simulink model "VVI"  (R2020a)
settings: Solver=FixedStepAuto  StartTime=0.0  StopTime=inf  FixedStep=0.001  RelTol=1e-3  EnableMultiTasking=on
undefined symbols (not defined in the file): D1, D10, D11, D12, D13, D2, D3, D4, D5, D7, D8, D9, PTA0, PTA1, PTA2, PTB23, PTB9, PTC17, PTC3, PTC4, PTD0, PTD1, PTD2, PTD3
libraries: frdmk64flib x12
settings Model: ExtModeTrigDuration=5  Creator=12268  LastModifiedBy=12268
settings OptimizationCC: EnhancedBackFolding=on  PassReuseOutputArgsAs=Individual arguments  ZeroExternalMemoryAtStartup=off  ZeroInternalMemoryAtStartup=off  MaxStackSize=64  OptimizeBlockOrder=speed  DifferentSizesBufferReuse=on  OptimizationCustomize=off  EfficientTunableParamExpr=on
settings DebuggingCC: ParameterTunabilityLossMsg=error
settings HardwareCC: ProdBitPerPointer=32  ProdBitPerSizeT=32  ProdBitPerPtrDiffT=32  ProdLargestAtomicInteger=Long  ProdLargestAtomicFloat=Double  ProdWordSize=32  ProdHWDeviceType=ARM Compatible->ARM Cortex
settings SFSimCC: MATLABDynamicMemAlloc=off
settings RTWCC: SystemTargetFile=ert.tlc  HardwareBoard=NXP FRDM-K64F  TemplateMakefile=ert_default_tmf  Toolchain=GNU Tools for ARM Embedded Processors
settings CodeAppCC: ForceParamTrailComments=on  IgnoreCustomStorageClasses=off  OperatorAnnotations=on  SimulinkDataObjDesc=on  SFDataObjDesc=on  InsertBlockDesc=on

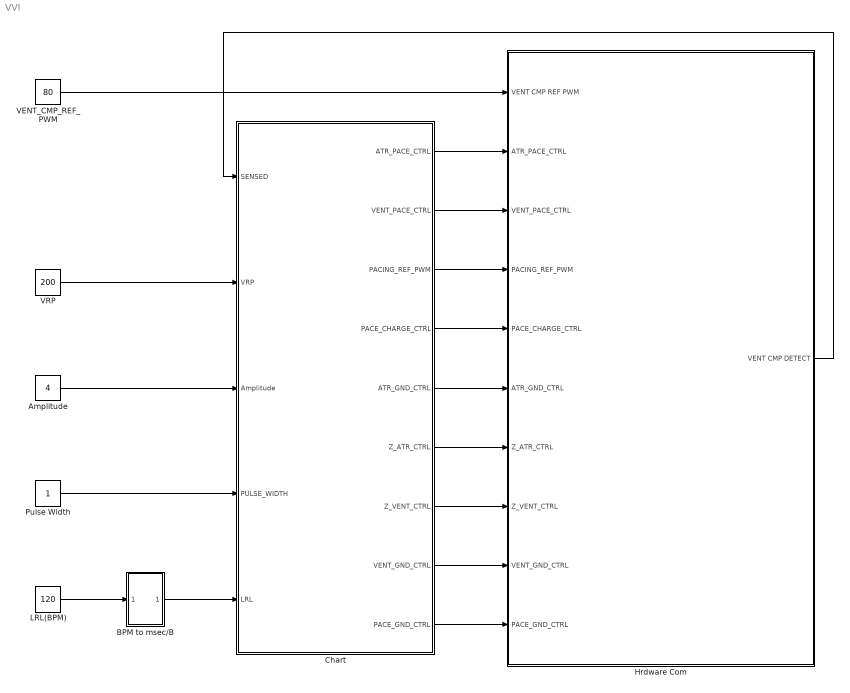
== system VVI ==
  Amplitude : Constant  Value=4  OutDataTypeStr=double
  "BPM to msec/B " : Subsystem
  Chart : Stateflow chart  TreatAsAtomicUnit=on
  Hrdware Com : Subsystem
  LRL(BPM) : Constant  Value=120  OutDataTypeStr=double
  Pulse Width : Constant  OutDataTypeStr=uint16
  VENT_CMP_REF_PWM : Constant  Value=80  OutDataTypeStr=double
  VRP : Constant  Value=200  OutDataTypeStr=uint16
  wires:
  Amplitude/1 -> Chart/3(Amplitude)
  LRL(BPM)/1 -> "BPM to msec/B "/1(In1)
  Pulse Width/1 -> Chart/4(PULSE_WIDTH)
  "BPM to msec/B "/1(Out1) -> Chart/5(LRL)
  Chart/1(ATR_PACE_CTRL) -> Hrdware Com/2(ATR_PACE_CTRL)
  Chart/2(VENT_PACE_CTRL) -> Hrdware Com/3(VENT_PACE_CTRL)
  Chart/3(PACING_REF_PWM) -> Hrdware Com/4(PACING_REF_PWM)
  Chart/4(PACE_CHARGE_CTRL) -> Hrdware Com/5(PACE_CHARGE_CTRL)
  Chart/5(ATR_GND_CTRL) -> Hrdware Com/6(ATR_GND_CTRL)
  Chart/6(Z_ATR_CTRL) -> Hrdware Com/7("Z_ATR_CTRL ")
  Chart/7(Z_VENT_CTRL) -> Hrdware Com/8("Z_VENT_CTRL ")
  Chart/8(VENT_GND_CTRL) -> Hrdware Com/9(VENT_GND_CTRL)
  Chart/9(PACE_GND_CTRL) -> Hrdware Com/10(PACE_GND_CTRL)
  Hrdware Com/1("VENT CMP DETECT ") -> Chart/1(SENSED)
  VENT_CMP_REF_PWM/1 -> Hrdware Com/1(VENT CMP REF PWM)
  VRP/1 -> Chart/2(VRP)

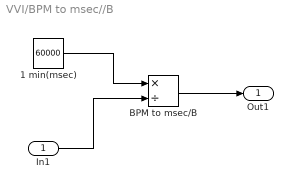
== system VVI/BPM to msec//B  ==
  In1 : Inport
  1 min(msec) : Constant  Value=60000  OutDataTypeStr=double
  "BPM to msec/B " : Product  Inputs=*/  OutDataTypeStr=uint16  RndMeth=Nearest
  Out1 : Outport
  wires:
  1 min(msec)/1 -> "BPM to msec/B "/1
  "BPM to msec/B "/1 -> Out1/1
  In1/1 -> "BPM to msec/B "/2

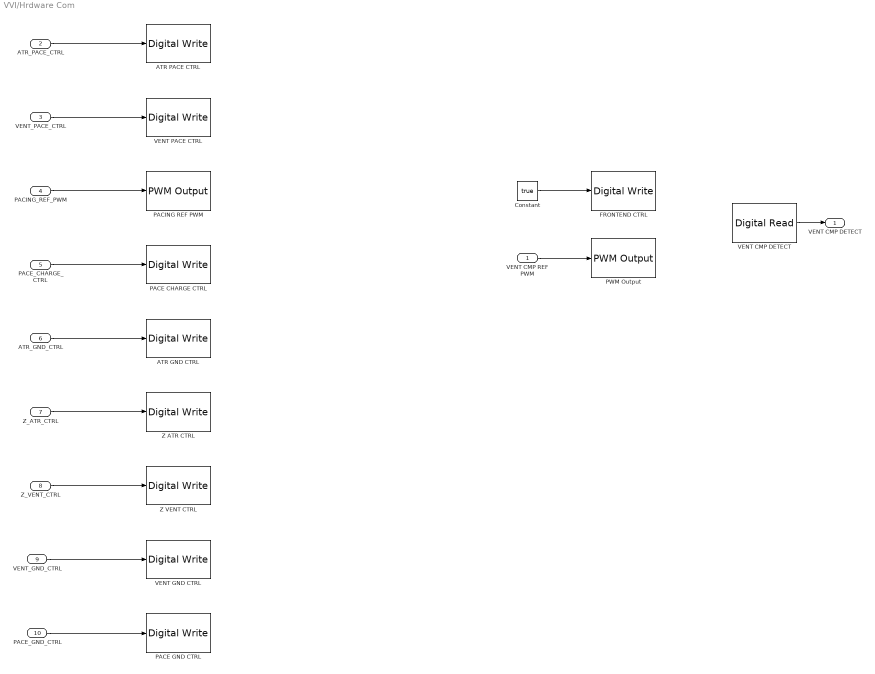
== system VVI/Hrdware Com ==
  VENT CMP REF PWM : Inport
  ATR_PACE_CTRL : Inport  Port=2
  VENT_PACE_CTRL : Inport  Port=3
  PACING_REF_PWM : Inport  Port=4
  PACE_CHARGE_CTRL : Inport  Port=5
  ATR_GND_CTRL : Inport  Port=6
  "Z_ATR_CTRL " : Inport  Port=7
  "Z_VENT_CTRL " : Inport  Port=8
  VENT_GND_CTRL : Inport  Port=9
  PACE_GND_CTRL : Inport  Port=10
  "ATR GND CTRL " : frdmk64flib/Digital Write  Whichpin=PTD2 (D11)
  ATR PACE CTRL : frdmk64flib/Digital Write  Whichpin=PTA0 (D8)
  Constant : Constant  Value=true  OutDataTypeStr=boolean
  FRONTEND CTRL : frdmk64flib/Digital Write  Whichpin=PTD1 (D13)
  PACE CHARGE CTRL : frdmk64flib/Digital Write  Whichpin=PTB9 (D2)
  PACE GND CTRL : frdmk64flib/Digital Write  Whichpin=PTD0 (D10)
  PACING REF PWM : frdmk64flib/PWM Output  Whichpin=PTA2 (D5)  InitialFrequency=2000  InitialDutyCycle=0
  PWM Output : frdmk64flib/PWM Output  Whichpin=PTA1 (D3)  InitialFrequency=2000  InitialDutyCycle=0
  VENT CMP DETECT : frdmk64flib/Digital Read  Whichpin=PTC17 (D1)  SampleTime=-1
  VENT GND CTRL : frdmk64flib/Digital Write  Whichpin=PTD3 (D12)
  VENT PACE CTRL : frdmk64flib/Digital Write  Whichpin=PTC4 (D9)
  "Z ATR CTRL " : frdmk64flib/Digital Write  Whichpin=PTB23 (D4)
  "Z VENT CTRL " : frdmk64flib/Digital Write  Whichpin=PTC3 (D7)
  "VENT CMP DETECT " : Outport  OutDataTypeStr=boolean  PortDimensions=1
  wires:
  ATR_PACE_CTRL/1 -> ATR PACE CTRL/1
  VENT_PACE_CTRL/1 -> VENT PACE CTRL/1
  PACING_REF_PWM/1 -> PACING REF PWM/1
  PACE_CHARGE_CTRL/1 -> PACE CHARGE CTRL/1
  ATR_GND_CTRL/1 -> "ATR GND CTRL "/1
  "Z_ATR_CTRL "/1 -> "Z ATR CTRL "/1
  "Z_VENT_CTRL "/1 -> "Z VENT CTRL "/1
  VENT_GND_CTRL/1 -> VENT GND CTRL/1
  PACE_GND_CTRL/1 -> PACE GND CTRL/1
  Constant/1 -> FRONTEND CTRL/1
  VENT CMP DETECT/1 -> "VENT CMP DETECT "/1
  VENT CMP REF PWM/1 -> PWM Output/1

== stateflow chart VVI/Chart ==
  state Charging_and_Discharging
    entry:
    PACE_GND_CTRL=true;
    ATR_PACE_CTRL=false;
    VENT_PACE_CTRL=false;
    PACING_REF_PWM=uint8(Amplitude*20);
    PACE_CHARGE_CTRL=true;
    Z_ATR_CTRL=false;
    Z_VENT_CTRL=false;
    ATR_GND_CTRL=false;
    VENT_GND_CTRL=true;
  state V_Pacing
    entry:
    PACE_CHARGE_CTRL=false;
    PACE_GND_CTRL=true;
    ATR_GND_CTRL=false;
    Z_ATR_CTRL=false;
    Z_VENT_CTRL=false;
    VENT_GND_CTRL=false;
    ATR_PACE_CTRL=false;
    VENT_PACE_CTRL=true;
    PACED=true;
  (junction 69) -> Charging_and_Discharging [order 1] : [SENSED==true]{PACED=false}
  (default) -> Charging_and_Discharging
  Charging_and_Discharging -> (junction 69) [order 2] : after(VRP, msec)[PACED==false]
  (junction 69) -> V_Pacing [order 2] : after(LRL-VRP, msec)
  (junction 70) -> V_Pacing [order 2] : after(LRL-VRP, msec)
  Charging_and_Discharging -> (junction 70) [order 1] : after(VRP-PULSE_WIDTH, msec)[PACED==true]
  (junction 70) -> Charging_and_Discharging [order 1] : [SENSED==true]{PACED=false}
  V_Pacing -> Charging_and_Discharging : after(PULSE_WIDTH, msec)
  data: SENSED input boolean; VRP input uint16; ATR_PACE_CTRL output boolean; VENT_PACE_CTRL output boolean; PACING_REF_PWM output uint8; Amplitude input double; PACE_CHARGE_CTRL output boolean; ATR_GND_CTRL output boolean; Z_ATR_CTRL output boolean; Z_VENT_CTRL output boolean; VENT_GND_CTRL output boolean; PACE_GND_CTRL output boolean; PULSE_WIDTH input uint16; LRL input uint16; PACED local boolean =false
